simulink model "quad_6DOF_quaternion_ANSFT"  (R2023a)
settings: Solver=ode1  StartTime=0.0  StopTime=10  FixedStep=0.01  RelTol=1e-3
libraries: sharedtransform x5, simulink_extras x4, matrix_library x3, aerolibutil x3, simulink x3, sharedutil x2, robotcorelib x1, uavutilslib x1
settings Model: Creator=adan  LastModifiedBy=Adan Daniel

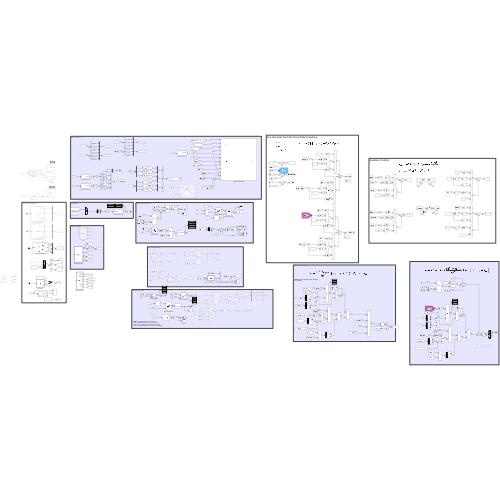
[thumbnail: Simulink's stored preview of the top-level diagram]
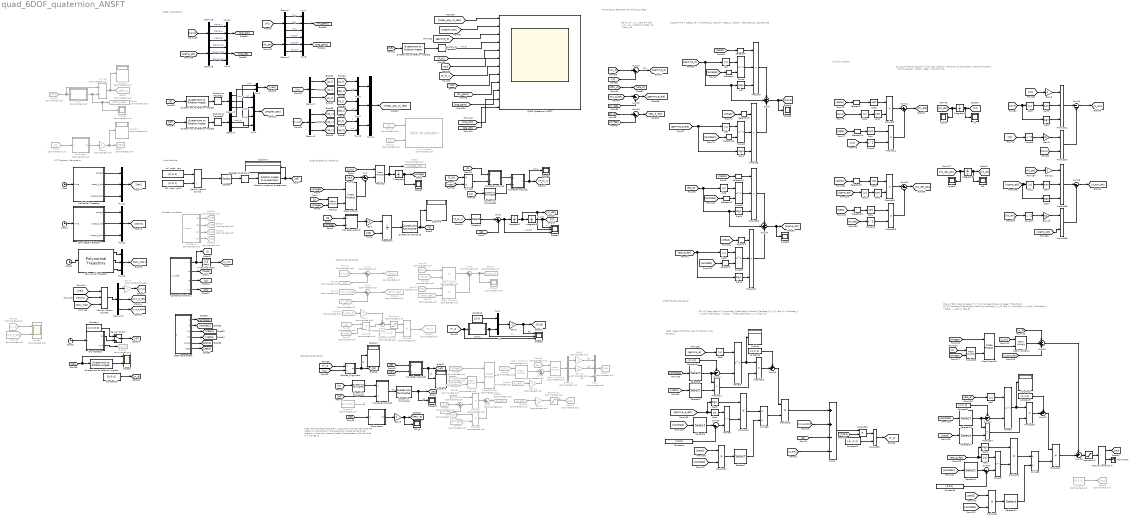
== system quad_6DOF_quaternion_ANSFT ==
  note: Note: It seems that the mass if missing in
      | the equation.
  note: ANSFT Position Controller
  note: $\tau = \Big [ \dot \omega_d + J^{-1} \omega \times J \omega + \frac{|\dot e|^{2-\lambda_2}\text{sign}(\dot e)}{\lambda_2 \xi_2} \Big (1 + \lambda_1 \xi_1|e|^{\lambda_1 - 1}\Big ) - u_{aux} \Big ]$
  note: $F_u = \frac{|\dot e|^{2-\lambda_2}\text{sign}(\dot e)}{\lambda_2 \xi_2} \Big (1 + \lambda_1 \xi_1|e|^{\lambda_1 - 1}\Big ) + \ddot \gamma_d - g - u_{aux}$
  note: Note : For the tilted Hexa-rotor I guess that I
      | have to calculate the vector nz, due to that in the
      | quad-rotor it used as the thrust direction in the body
      | frame of itself. Nonetheless in the FAH that will change ig
  note: Attitude PD Controller
  note: Initial attitude
  note: Constant variables
  note: Data Visualization
  note: Position PD Controller
  note: Quad Quaternion Modeling
  note: XYZ Trajectory Generation
  note: $e = x_d - x_1 \\ \dot e = \dot x_d - x_2 \\ \ddot e = \ddot x_d - \dot x_2$
  note: $\sigma = e + \zeta_1 |e| ^{\lambda_1} sign(e) + \zeta_2 | \dot e| ^{\lambda_2} sign(\dot e)$
  note: Non-Singular Fast Terminal Sliding Surface
  note: Auxiliary Control
  note: $u_{aux}=-2K(t) |\sigma|^{1/2} sign (\sigma) - \frac{K(t)^2}{2}\sigma \\ \dot K(t) = \alpha ^{1/2} |\sigma| ^{1/2} - \beta ^{1/2}K(t)^2$
  ANSFT parameters : MATLAB Function  TreatAsAtomicUnit=on
  Abs{,1..11} (12 alike) : Abs  SaturateOnIntegerOverflow=off
  Attitude_Alignment : Subsystem
  Clock{,1..3} (4 alike) : Clock
  Constant : Constant  Value=[1; 0; 0; 0]
  Constant1 : Constant  Value=[0; 0]
  Constant10 : Constant  Value=[0; 0; 0]
  Constant11 : Constant  Value=[-1; -1; 1]
  Constant2 : Constant  Commented=on  Value=[1; 0; 0; 0]
  Constant{3,5,7,9} (4 alike) : Constant  Value=[1; 1; 1]
  Constant4 : Constant  Value=[2;2;2]
  Constant6 : Constant  Commented=on  Value=[0; 0; 0]
  Constant8 : Constant  Value=[2;2;2]
  Constants Functions : MATLAB Function  TreatAsAtomicUnit=on
  Cross Product : matrix_library/Cross Product
  Cross Product1 : matrix_library/Cross Product
  Cross Product2 : matrix_library/Cross Product  Commented=on
  Degrees to Radians : simulink_extras/Transformations/Degrees to Radians
  Demux{1..4,6..9,11} (9 alike) : Demux  Outputs=3
  Demux5 : Demux  Commented=on  Outputs=3
  Display{,3..7} (6 alike) : Display
  Display1 : Display  Commented=on
  Display2 : Display  Commented=on
  Divide : Product  Commented=on  Inputs=*/
  Divide1 : Product  Inputs=*/
  Divide2 : Product  Inputs=*/
  Divide3 : Product  Inputs=*/
  Force adjustment : Constant  Commented=on  Value=[-1; -1; 1]
  From10 : From  Commented=on  GotoTag=PRP
  From12 : From  Commented=on  GotoTag=q
  From18 : From  Commented=on  GotoTag=xi
  From19 : From  Commented=on  GotoTag=kpt
  From20 : From  Commented=on  GotoTag=kdt
  From23 : From  Commented=on  GotoTag=xyz_d
  From24 : From  Commented=on  GotoTag=xyz_d_dot
  From26 : From  Commented=on  GotoTag=xi_dot
  From27 : From  Commented=on  GotoTag=xi
  From28 : From  Commented=on  GotoTag=error
  From29 : From  Commented=on  GotoTag=error_dot
  From30 : From  Commented=on  GotoTag=xyz_d
  From31 : From  Commented=on  GotoTag=g
  From44 : From  Commented=on  GotoTag=u_aux_z
  From46 : From  Commented=on  GotoTag=xyz_d_dot
  From47 : From  Commented=on  GotoTag=mass
  From56 : From  Commented=on  GotoTag=J_inv
  From57 : From  Commented=on  GotoTag=J
  From58 : From  Commented=on  GotoTag=omega
  From59 : From  Commented=on  GotoTag=omega
  From60 : From  Commented=on  GotoTag=PRV_e
  From61 : From  Commented=on  GotoTag=kdr
  From62 : From  Commented=on  GotoTag=omega
  From63 : From  Commented=on  GotoTag=kpr
  From64 : From  Commented=on  GotoTag=u_aux
  From65 : From  Commented=on  GotoTag=J
  From66 : From  Commented=on  GotoTag=u_aux
  From9 : From  Commented=on  GotoTag=q
  From90 : From  Commented=on  GotoTag=w_d
  Gain : Gain  Gain=0.5
  Gain1 : Gain  Commented=on  Gain=2
  Gain{4,7,9..11} (5 alike) : Gain  Commented=on  Gain=-1
  Gain12 : Gain  Gain=2
  Gain13 : Gain  Gain=0.5
  Gain2 : Gain  Gain=-1
  Gain3 : Gain  Gain=2
  Gain5 : Gain  Commented=through  Gain=0
  Gain6 : Gain  Gain=2
  Gain8 : Gain  Gain=0.5
  Goto13 : Goto  Commented=on  GotoTag=F_u
  Goto16 : Goto  Commented=on  GotoTag=kpt
  Goto17 : Goto  Commented=on  GotoTag=kdt
  Goto19 : Goto  Commented=on  GotoTag=kpr
  Goto20 : Goto  Commented=on  GotoTag=kdr
  Goto21 : Goto  Commented=on  GotoTag=error
  Goto22 : Goto  Commented=on  GotoTag=error_dot
  Goto29 : Goto  Commented=on  GotoTag=tau
  Goto3 : Goto  Commented=on  GotoTag=omega_dot
  Goto30 : Goto  Commented=on  GotoTag=u_aux
  Goto31 : Goto  Commented=on  GotoTag=u_aux_z
  Goto37 : Goto  Commented=on  GotoTag=tau
  Goto49 : Goto  Commented=on  GotoTag=w_d
  Goto59 : Goto  Commented=on  GotoTag=tau
  Goto6 : Goto  Commented=on  GotoTag=PRP
  Goto8 : Goto  Commented=on  GotoTag=PRP_u
  Goto9 : Goto  Commented=on  GotoTag=PRP_angle
  Helicoidal Trajectory : MATLAB Function  TreatAsAtomicUnit=on
  Integrator : Integrator  InitialCondition=[0; 0; 0]
  Integrator1 : Integrator  InitialConditionSource=external
  Integrator2 : Integrator  InitialCondition=[0; 0; 0]
  Integrator3 : Integrator  InitialCondition=[0; 0; 0]
  Integrator4 : Integrator  InitialCondition=[0;0;0]
  Integrator5 : Integrator  InitialCondition=[0;0;0]
  Invert 3x3 Matrix : aerolibutil/Invert  3x3 Matrix
  Kronecker product : Subsystem
  Kronecker product1 : Subsystem
  Kronecker product2 : Subsystem
  Kronecker product3 : Subsystem
  Kronecker product4 : Subsystem
  Kt : Scope
  Kt1 : Scope
  Kt_dot : Scope
  Kt_dot1 : Scope
  Lemniscate Trajectory : MATLAB Function  TreatAsAtomicUnit=on
  Manual Variant Sink : simulink/Signal Routing/Manual Variant Sink  NumChoices=2  LabelModeActiveChoice=V_1
  Manual Variant Source : simulink/Signal Routing/Manual Variant Source  NumChoices=2  LabelModeActiveChoice=V_1
  Manual Variant Source1 : simulink/Signal Routing/Manual Variant Source  NumChoices=3  LabelModeActiveChoice=V_3
  Manual Switch : ManualSwitch
  Matrix Multiply : Product  Commented=on
  Matrix Multiply1 : Product  Commented=on
  Matrix Multiply2 : Product  Multiplication=Matrix(*)
  Matrix Multiply3 : Product  Commented=on  Multiplication=Matrix(*)
  Matrix Multiply4 : Product  Commented=on  Multiplication=Matrix(*)
  Mux{1,3,8..10} (5 alike) : Mux  Inputs=2
  Mux{5..7,11..12,21..23} (8 alike) : Mux  Inputs=3
  Mux2 : Mux
  Mux4 : Mux  Commented=on  Inputs=3
  PD Gains : MATLAB Function  Commented=on  TreatAsAtomicUnit=on
  PRV_e : Scope
  Polynomial Trajectory : robotcorelib/Polynomial Trajectory  WaypointSource=Internal  Waypoints=[0, 0, 0, 0, 0, 0; 0, 0, 0, 0, 0, 0; 0, -2, -4, -4, -2, 0]*0  TimePoints=[ 0, 12, 24, 36, 48, 60]  TimeInterval=[ 1, 4 ]  Method=Cubic Polynomial  ParameterSource=Internal  VelocityBoundaryCondition=zeros( 3, 6)  AccelerationBoundaryCondition=zeros( 2, 5 )  SimulateUsing=Interpreted execution
  Power{,1,4..9} (8 alike) : Math  Operator=pow
  Power{2..3,10..11} (4 alike) : Math  Operator=square
  Product : Product  Multiplication=Matrix(*)
  Product1 : Product  Multiplication=Matrix(*)
  Product{9..11,13..18,20..25,28..29,31} (18 alike) : Product
  Product{4,8,12,26..27,30} (6 alike) : Product  Inputs=3
  Product19 : Product  Multiplication=Matrix(*)
  Product{2..3,6..7} (4 alike) : Product  Commented=on
  Product5 : Product  Commented=on  Multiplication=Matrix(*)
  QUAD Quaternion ANSFT : Scope  NumInputPorts=12
  Quaternion Conjugate : aerolibutil/Quaternion Conjugate
  Quaternion Conjugate2 : aerolibutil/Quaternion Conjugate
  Quaternion Normalize : sharedutil/Quaternion Normalize  aMode=aMode
  Quaternion Normalize1 : sharedutil/Quaternion Normalize  aMode=aMode
  Quaternions to Rotation Angles1 : sharedtransform/Quaternions to Rotation Angles  rotationOrder=ZYX  aMode=aMode
  Quaternions to Rotation Angles2 : sharedtransform/Quaternions to Rotation Angles  rotationOrder=XYZ  aMode=aMode
  Quaternions to Rotation Angles3 : sharedtransform/Quaternions to Rotation Angles  rotationOrder=ZYX  aMode=aMode
  Quaternions to Rotation Angles4 : sharedtransform/Quaternions to Rotation Angles  rotationOrder=ZYX  aMode=aMode
  Radians to Degrees1 : simulink_extras/Transformations/Radians to Degrees
  Radians to Degrees2 : simulink_extras/Transformations/Radians to Degrees
  Radians to Degrees3 : simulink_extras/Transformations/Radians to Degrees
  Rotation Angles to Quaternions : sharedtransform/Rotation Angles to Quaternions  rotationOrder=ZYX  aMode=aMode
  Saturation : Saturate  Commented=on  UpperLimit=[2; 2; 0]  LowerLimit=[-2; -2; -28]
  Saturation1 : Saturate  Commented=on
  Saturation2 : Saturate
  Scope : Scope  Commented=on
  Scope1 : Scope  NumInputPorts=2
  Scope{3,7..10} (5 alike) : Scope
  Scope2 : Scope  NumInputPorts=3
  Scope4 : Scope  NumInputPorts=3
  Scope5 : Scope  Commented=on
  Scope6 : Scope  Commented=on  NumInputPorts=2
  Selector : Selector  InputPortWidth=3  IndexOptions=Index vector (dialog)  Indices=[3 2 1]  OutputSizes=1
  Selector{1,3,10..14,18,20..21} (10 alike) : Selector  InputPortWidth=6  IndexOptions=Index vector (dialog)  Indices=[4:6]  OutputSizes=1
  Selector{4..9,15..17,19} (10 alike) : Selector  InputPortWidth=6  IndexOptions=Index vector (dialog)  Indices=[1:3]  OutputSizes=1
  Selector2 : Selector  InputPortWidth=4  IndexOptions=Index vector (dialog)  Indices=[2:4]  OutputSizes=1
  Sign{,1..7} (8 alike) : Signum
  Sqrt{,1..7} (8 alike) : Sqrt
  Subsystem : Subsystem  Commented=on
  Subsystem1 : Subsystem
  Sum{,11,14..16,25} (6 alike) : Sum  Inputs=|+-
  Sum1 : Sum  Inputs=|++
  Sum10 : Sum  Inputs=|-+
  Sum12 : Sum  Inputs=|--
  Sum13 : Sum  Commented=on  Inputs=|+-
  Sum17 : Sum  Inputs=-+|
  Sum18 : Sum  Inputs=++|
  Sum19 : Sum  Inputs=++-
  Sum2 : Sum  Commented=on  Inputs=|+-
  Sum20 : Sum  Inputs=|-+
  Sum21 : Sum  Inputs=-+|
  Sum22 : Sum  Inputs=++|
  Sum23 : Sum  Inputs=++|
  Sum24 : Sum  Inputs=+++
  Sum26 : Sum  Inputs=|--
  Sum3 : Sum  Commented=on  Inputs=|+-
  Sum4 : Sum  Commented=on  Inputs=|++
  Sum5 : Sum  Commented=on  Inputs=+-|
  Sum6 : Sum  Inputs=++--
  Sum7 : Sum  Commented=on  Inputs=|++
  Sum8 : Sum  Commented=on  Inputs=|++
  Sum9 : Sum  Inputs=+++
  Terminator : Terminator
  UAV Animation : uavutilslib/UAV Animation  Commented=on  UAVType=Multirotor  UAVSize=1  InertialZDirection=Down  SampleTime=-1
  Yaw trajectory : MATLAB Function  TreatAsAtomicUnit=on
  norm : MATLAB Function  Commented=on  TreatAsAtomicUnit=on
  norm1 : MATLAB Function  TreatAsAtomicUnit=on
  "roll, pitch, yaw" : Constant  Value=[5; 0; 0]
  "roll, pitch, yaw1" : Constant  Value=[0; 0; 1]
  wires:
  Constants Functions/1(J) -> [J], Invert 3x3 Matrix/1
  Invert 3x3 Matrix/1 -> [J_inv]
  [tau] -> Sum/1
  [J] -> Product/1
  [omega] -> Product/2
  [omega] -> Cross Product/1
  Product/1 -> Cross Product/2
  Cross Product/1 -> Sum/2
  Sum/1 -> Product1/2
  [J_inv] -> Product1/1
  Product1/1 -> Goto3/1, Integrator/1
  Integrator/1 -> Scope7/1, [omega]
  [omega] -> Kronecker product/2(p)
  Kronecker product/1(r) -> Gain/1
  Gain/1 -> Integrator1/1
  Degrees to Radians/1 -> Rotation Angles to Quaternions/1
  Selector/1 -> Degrees to Radians/1
  Rotation Angles to Quaternions/1 -> Display4/1, [q0]
  [q0] -> Integrator1/2
  Integrator1/1 -> Quaternion Normalize/1
  [q] -> Kronecker product/1(q)
  Quaternion Normalize/1 -> Display5/1, [q]
  From12/1 -> UAV Animation/2
  From18/1 -> UAV Animation/1
  Constants Functions/2(m) -> [mass]
  From9/1 -> Subsystem/1(q)
  Subsystem/1(lnq) -> Gain1/1
  Gain1/1 -> Display1/1, Goto6/1
  From10/1 -> norm/1(u), Divide/1
  norm/1(y) -> Scope/1, Goto9/1, Divide/2
  Divide/1 -> Goto8/1, Display2/1
  Constants Functions/3(g) -> [g]
  Kronecker product1/1(r) -> Kronecker product2/1(q)
  Kronecker product2/1(r) -> Scope3/1, [F_th_I]  "f_th_I"
  [F_th_I] -> Selector2/1
  [mass] -> Divide1/2
  Selector2/1 -> Sum1/1
  [g] -> Sum1/2
  Sum1/1 -> Scope4/3, Integrator2/1  "x_ddot"
  Integrator2/1 -> Scope4/2, [xi_dot], Integrator3/1  "x_dot"
  Integrator3/1 -> Scope4/1, [xi]  "x"
  PD Gains/1(kpt) -> Goto16/1
  PD Gains/2(kdt) -> Goto17/1
  PD Gains/4(kdr) -> Goto20/1
  PD Gains/3(kpr) -> Goto19/1
  Polynomial Trajectory/3 -> Mux23/3
  Mux22/1 -> [lemni]
  Clock1/1 -> Polynomial Trajectory/1
  Manual Variant Source1/1 -> Demux11/1
  Demux11/2 -> [xyz_d_dot]
  Mux21/1 -> [heli]
  Helicoidal Trajectory/1(pose_d) -> Mux21/1
  Lemniscate Trajectory/2(pose_d_dot) -> Mux22/2
  [lemni] -> Manual Variant Source1/2
  Clock2/1 -> Lemniscate Trajectory/1(time)
  [poly_tray] -> Manual Variant Source1/3
  Helicoidal Trajectory/3(pose_d_ddot) -> Mux21/3
  [heli] -> Manual Variant Source1/1
  Lemniscate Trajectory/3(pose_d_ddot) -> Mux22/3
  Mux23/1 -> [poly_tray]
  Clock/1 -> Helicoidal Trajectory/1(time)
  Polynomial Trajectory/2 -> Mux23/2
  Polynomial Trajectory/1 -> Mux23/1
  Helicoidal Trajectory/2(pose_d_dot) -> Mux21/2
  Demux11/3 -> [xyz_d_ddot]
  Demux11/1 -> Gain5/1
  Lemniscate Trajectory/1(pose_d) -> Mux22/1
  From23/1 -> Sum2/1
  From27/1 -> Sum2/2
  From24/1 -> Sum3/1
  From26/1 -> Sum3/2
  Sum2/1 -> Goto21/1
  Sum3/1 -> Goto22/1
  From19/1 -> Matrix Multiply/1
  From28/1 -> Matrix Multiply/2
  From20/1 -> Matrix Multiply1/1
  From29/1 -> Matrix Multiply1/2
  Matrix Multiply/1 -> Sum4/1
  Matrix Multiply1/1 -> Sum4/2
  Sum5/1 -> Saturation/1
  [F_u] -> norm1/1(u), Scope2/3  "fu"
  norm1/1(y) -> Mux1/2, Scope2/2  "nu"
  Constant1/1 -> Mux1/1
  Mux1/1 -> Gain2/1
  Gain2/1 -> [F_th], Scope2/1  "fth"
  [angular_pos] -> QUAD Quaternion ANSFT/2
  [gamma_e] -> QUAD Quaternion ANSFT/3
  Quaternions to Rotation Angles2/1 -> Radians to Degrees2/1
  [F_th_I] -> QUAD Quaternion ANSFT/7
  [yaw] -> QUAD Quaternion ANSFT/8
  [tau] -> QUAD Quaternion ANSFT/6
  [F_th] -> QUAD Quaternion ANSFT/5
  [linear_pos_vs_des] -> QUAD Quaternion ANSFT/1
  [q_x] -> Mux8/1  "x"
  [qd_y] -> Mux9/2  "y_d"
  Mux8/1 -> Mux11/1
  Mux9/1 -> Mux11/2
  [qd_x] -> Mux8/2  "x_d"
  Mux11/1 -> [linear_pos_vs_des]
  [q_y] -> Mux9/1  "y"
  Mux10/1 -> Mux11/3
  [qd_z] -> Mux10/2  "z_d"
  [q_z] -> Mux10/1  "z"
  Demux6/3 -> [qd_z]
  [xyz_d] -> Demux6/1
  Demux6/2 -> [qd_y]
  Demux6/1 -> [qd_x]
  Demux2/1 -> [q_x]
  Demux2/2 -> [q_y]
  Demux2/3 -> [q_z]
  [xi] -> Demux2/1
  [q] -> Quaternions to Rotation Angles1/1
  Subsystem1/1(lnq) -> Gain3/1
  Clock3/1 -> Yaw trajectory/1(t)
  [qz] -> Kronecker product3/2(p)
  Kronecker product3/1(r) -> Display6/1, [qd]  "qd"
  [q] -> Quaternion Conjugate/1
  Quaternion Conjugate/1 -> Kronecker product4/1(q)
  Kronecker product4/1(r) -> Quaternion Normalize1/1  "qe"
  Gain3/1 -> PRV_e/1, [PRV_e]
  Constants Functions/4(nz) -> [nz]
  [F_u] -> Attitude_Alignment/1(nu)
  [nz] -> Attitude_Alignment/2(nz)
  Attitude_Alignment/1(qt) -> Display7/1, [qt]  "qt"
  [qe] -> Quaternions to Rotation Angles2/1
  [qd] -> Quaternions to Rotation Angles3/1
  Quaternions to Rotation Angles1/1 -> Radians to Degrees1/1
  Demux3/1 -> Mux3/1  "yaw"
  Demux3/2 -> Mux2/3  "pitch"
  Demux3/3 -> Mux2/1  "roll"
  Demux4/1 -> Mux3/2  "yaw_d"
  Demux4/3 -> Mux2/2  "roll_d"
  Demux4/2 -> Mux2/4  "pitch_d"
  Quaternions to Rotation Angles3/1 -> Radians to Degrees3/1
  [qz] -> Scope1/1, Quaternions to Rotation Angles4/1
  Quaternions to Rotation Angles4/1 -> Scope1/2
  Yaw trajectory/1(qz) -> Manual Switch/2
  Constant/1 -> Manual Switch/1
  Manual Switch/1 -> [qz]
  From58/1 -> Product5/2
  Product5/1 -> Cross Product2/2
  From57/1 -> Product5/1
  From59/1 -> Cross Product2/1
  Cross Product2/1 -> Matrix Multiply3/2
  From56/1 -> Matrix Multiply3/1
  From62/1 -> Sum13/2
  From61/1 -> Product7/1
  Product7/1 -> Sum7/1
  From63/1 -> Product6/1
  From60/1 -> Product6/2
  Product6/1 -> Sum7/2
  Sum7/1 -> Goto30/1
  Matrix Multiply3/1 -> Sum8/1
  From64/1 -> Gain11/1
  Sum8/1 -> Matrix Multiply4/2
  From65/1 -> Matrix Multiply4/1
  Matrix Multiply4/1 -> Demux5/1
  Mux2/1 -> [angular_pos]
  Radians to Degrees2/1 -> QUAD Quaternion ANSFT/4  "rpy_e"
  Sum4/1 -> Scope5/1, Goto31/1
  From44/1 -> Gain4/1
  Radians to Degrees1/1 -> Demux3/1
  Radians to Degrees3/1 -> Demux4/1
  [qe] -> Subsystem1/1(q)
  Saturation/1 -> Product3/1
  Gain4/1 -> Sum5/1
  [q] -> Quaternion Conjugate2/1
  [q] -> Kronecker product1/1(q)
  From30/1 -> Scope6/1
  From46/1 -> Scope6/2
  Product2/1 -> Sum5/2
  From31/1 -> Product2/1
  From47/1 -> Product2/2
  Gain5/1 -> [xyz_d]
  [F_th] -> Divide1/1
  [qd] -> Kronecker product4/2(p)
  From66/1 -> Gain7/1
  Quaternion Conjugate2/1 -> Kronecker product2/2(p)
  Manual Variant Source/1 -> Selector/1
  "roll, pitch, yaw"/1 -> Manual Variant Source/1
  "roll, pitch, yaw1"/1 -> Manual Variant Source/2
  Saturation1/1 -> Goto37/1  "tau"
  Force adjustment/1 -> Product3/2
  Product3/1 -> Goto13/1
  Gain7/1 -> Saturation1/1
  Quaternion Normalize1/1 -> Scope10/1, [qe]  "qe"
  Mux3/1 -> [yaw]
  [zeta1] -> Selector4/1
  Sign/1 -> Product4/3
  Power1/1 -> Product8/2
  [gamma_e] -> Sum9/2, Sign/1, Abs/1
  Product8/1 -> Sum9/3
  Abs1/1 -> Power1/1
  [zeta2] -> Selector15/1
  Sign1/1 -> Product8/3
  [lambda1] -> Selector5/1
  [lambda2] -> Selector16/1
  Power/1 -> Product4/2
  Sum9/1 -> Scope9/1, [sigma]
  Product4/1 -> Sum9/1
  [gamma_e_dot] -> Sign1/1, Abs1/1
  Abs/1 -> Power/1
  Power2/1 -> Product11/2
  Product10/1 -> Sum12/2
  [Kt] -> Gain6/1
  Power3/1 -> Gain8/1
  Sum11/1 -> [Kt_dot]
  Product9/1 -> Sum11/1
  [Kt_dot] -> Kt_dot/1, Integrator4/1
  [sigma] -> Sign2/1, Abs3/1
  [alpha] -> Selector17/1
  Sqrt/1 -> Product11/1
  Sqrt1/1 -> Product9/1
  [Kt] -> Power2/1
  [beta] -> Selector19/1
  Product11/1 -> Sum11/2
  Gain6/1 -> Product12/1
  Abs3/1 -> Sqrt3/1
  Abs2/1 -> Sqrt2/1
  [Kt] -> Power3/1
  Gain8/1 -> Product10/1
  Sign2/1 -> Product12/3
  Sqrt2/1 -> Product9/2
  Sqrt3/1 -> Product12/2
  Sum12/1 -> [u_aux]
  Product12/1 -> Sum12/1
  [sigma] -> Product10/2
  Integrator4/1 -> Kt/1, [Kt]
  Divide1/1 -> Kronecker product1/2(p)
  [qt] -> Kronecker product3/1(q)
  Demux5/1 -> Gain9/1
  Gain9/1 -> Mux4/1  "t_x"
  Demux5/2 -> Gain10/1
  Demux5/3 -> Mux4/3  "t_z"
  Mux4/1 -> Goto29/1
  Gain10/1 -> Mux4/2  "t_y"
  Gain11/1 -> Sum8/2
  Yaw trajectory/2(w_d) -> Goto49/1
  From90/1 -> Sum13/1
  Sum13/1 -> Product7/2
  [xi] -> Sum14/2
  [w_d] -> Sum16/1
  [xi_dot] -> Sum15/2
  [omega] -> Sum16/2
  [xyz_d] -> Sum14/1
  [xyz_d_dot] -> Sum15/1
  ANSFT parameters/1(lambda1) -> [lambda1]
  ANSFT parameters/4(xi2) -> [zeta2]
  ANSFT parameters/2(lambda2) -> [lambda2]
  ANSFT parameters/3(xi1) -> [zeta1]
  ANSFT parameters/6(beta) -> [beta]
  ANSFT parameters/5(alpha) -> [alpha]
  [xyz_d_ddot] -> Sum6/2
  [g] -> Sum6/3
  [u_aux] -> Sum6/4
  [gamma_e_dot] -> Sign3/1, Abs4/1
  [lambda2] -> Selector6/1
  Constant4/1 -> Sum10/2
  Sum10/1 -> Power4/2
  Abs4/1 -> Power4/1
  Selector6/1 -> Sum10/1
  Sign3/1 -> Product13/1
  Power4/1 -> Product13/2
  Product13/1 -> Divide2/1
  [lambda2] -> Product14/2
  [zeta2] -> Product14/1
  Product14/1 -> Selector7/1
  Selector7/1 -> Divide2/2
  Divide2/1 -> Product15/2
  [gamma_e] -> Abs5/1
  Abs5/1 -> Power5/1
  Sum17/1 -> Power5/2
  [lambda1] -> Selector8/1
  Selector8/1 -> Product17/1, Sum17/2
  Constant3/1 -> Sum17/1
  Power5/1 -> Display/1, Product16/1
  Selector9/1 -> Product17/2
  [zeta1] -> Selector9/1
  Product17/1 -> Product16/2
  Sum18/1 -> Product15/1
  Product16/1 -> Sum18/2
  Constant5/1 -> Sum18/1
  Product15/1 -> Sum6/1
  Constant6/1 -> Goto59/1
  Constant2/1 -> ?
  Sum6/1 -> Product18/1
  [Kt] -> Demux7/1
  Mux7/1 -> [lin_gains]
  Demux7/3 -> Mux7/3  "Kt_z"
  Demux7/2 -> Mux7/2  "Kt_y"
  Demux7/1 -> Mux7/1  "Kt_x"
  [lin_gains] -> QUAD Quaternion ANSFT/9
  [ang_gains] -> QUAD Quaternion ANSFT/10
  [mass] -> Product18/2
  [J] -> Product19/1
  Cross Product1/1 -> Matrix Multiply2/2
  [omega] -> Cross Product1/1
  [J_inv] -> Matrix Multiply2/1
  [omega] -> Product19/2
  Product19/1 -> Cross Product1/2
  Matrix Multiply2/1 -> Sum19/2
  [u_aux_att] -> Sum19/3
  [w_d] -> Sum19/1
  Selector14/1 -> Product24/2
  Power6/1 -> Product20/2
  Constant7/1 -> Sum21/1
  Product21/1 -> Selector12/1
  [lambda2] -> Product21/2
  Product23/1 -> Sum22/2
  Selector12/1 -> Divide3/2
  [zeta1] -> Selector14/1
  Product20/1 -> Divide3/1
  Constant9/1 -> Sum22/1
  Sum21/1 -> Power7/2
  Sum22/1 -> Product22/1
  [lambda2] -> Selector11/1
  Sign4/1 -> Product20/1
  Sum20/1 -> Power6/2
  Selector11/1 -> Sum20/1
  Constant8/1 -> Sum20/2
  [zeta2] -> Product21/1
  Power7/1 -> Display3/1, Product23/1
  Abs7/1 -> Power7/1
  Selector13/1 -> Product24/1, Sum21/2
  [lambda1] -> Selector13/1
  Abs6/1 -> Power6/1
  [eta_e] -> Abs7/1
  Product24/1 -> Product23/2
  [eta_e_dot] -> Sign4/1, Abs6/1
  Divide3/1 -> Product22/2
  Product22/1 -> Sum23/2
  Sum23/1 -> Saturation2/1
  Sum19/1 -> Sum23/1
  Constant10/1 -> [w_d]
  Product18/1 -> Product25/1
  Constant11/1 -> Product25/2
  Product25/1 -> [F_u]
  Saturation2/1 -> Manual Variant Sink/1
  Manual Variant Sink/1 -> [tau]
  Manual Variant Sink/2 -> Terminator/1
  Sum15/1 -> [gamma_e_dot]
  Sum14/1 -> [gamma_e]  "des"
  Sum16/1 -> [eta_e_dot]
  [PRV_e] -> [eta_e]
  Selector4/1 -> Product4/1
  Selector5/1 -> Power/2
  Selector15/1 -> Product8/1
  Selector16/1 -> Power1/2
  Selector17/1 -> Sqrt1/1
  [sigma] -> Abs2/1
  Selector19/1 -> Sqrt/1
  Selector18/1 -> Power8/2
  Selector10/1 -> Product26/1
  Selector3/1 -> Power9/2
  Product26/1 -> Sum24/1
  Abs8/1 -> Power8/1
  Power9/1 -> Product27/2
  Power8/1 -> Product26/2
  [eta_e_dot] -> Abs9/1, Sign6/1
  [eta_e] -> Sum24/2, Sign5/1, Abs8/1
  Selector1/1 -> Product27/1
  [lambda1] -> Selector18/1
  Sign6/1 -> Product27/3
  Abs9/1 -> Power9/1
  Product27/1 -> Sum24/3
  Sign5/1 -> Product26/3
  Sum24/1 -> Scope8/1, [sigma_att]
  [lambda2] -> Selector3/1
  [zeta2] -> Selector1/1
  [zeta1] -> Selector10/1
  Selector21/1 -> Sqrt4/1
  Product30/1 -> Sum26/1
  Sqrt7/1 -> Product30/2
  Sqrt4/1 -> Product29/1
  Selector20/1 -> Sqrt5/1
  [sigma_att] -> Sign7/1, Abs11/1
  [beta] -> Selector21/1
  [Kt_att] -> Power10/1
  Sign7/1 -> Product30/3
  [sigma_att] -> Abs10/1
  Gain13/1 -> Product28/1
  Integrator5/1 -> Kt1/1, [Kt_att]
  Abs10/1 -> Sqrt6/1
  Power11/1 -> Gain13/1
  Product28/1 -> Sum26/2
  Power10/1 -> Product29/2
  [alpha] -> Selector20/1
  Product31/1 -> Sum25/1
  Sqrt5/1 -> Product31/1
  [Kt_att] -> Power11/1
  [sigma_att] -> Product28/2
  Sqrt6/1 -> Product31/2
  Product29/1 -> Sum25/2
  [Kt_dot_att] -> Kt_dot1/1, Integrator5/1
  Abs11/1 -> Sqrt7/1
  Sum26/1 -> [u_aux_att]
  Sum25/1 -> [Kt_dot_att]
  [Kt_att] -> Gain12/1
  Gain12/1 -> Product30/1
  Demux1/2 -> Mux5/2  "Kt_pitch"
  Demux1/3 -> Mux5/3  "Kt_yaw"
  Mux5/1 -> [ang_gains]
  Demux1/1 -> Mux5/1  "Kt_roll"
  [Kt_att] -> Demux1/1
  Demux8/2 -> Mux6/2  "sigma_pitch"
  Demux8/3 -> Mux6/3  "sigma_yaw"
  [sigma_att] -> Demux8/1
  Demux9/2 -> Mux12/2  "sigma_y"
  Demux9/3 -> Mux12/3  "sigma_z"
  Demux9/1 -> Mux12/1  "sigma_x"
  Demux8/1 -> Mux6/1  "sigma_roll"
  [sigma] -> Demux9/1
  Mux12/1 -> [sig_pos]
  Mux6/1 -> [sig_att]
  [sig_pos] -> QUAD Quaternion ANSFT/11
  [sig_att] -> QUAD Quaternion ANSFT/12

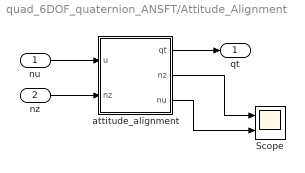
== system quad_6DOF_quaternion_ANSFT/Attitude_Alignment ==
  nu : Inport
  nz : Inport  Port=2
  Scope : Scope  NumInputPorts=2
  attitude_alignment : MATLAB Function  TreatAsAtomicUnit=on
  qt : Outport
  wires:
  attitude_alignment/1(qt) -> qt/1
  nz/1 -> attitude_alignment/2("nz ")
  nu/1 -> attitude_alignment/1(u)
  attitude_alignment/2(nz) -> Scope/1
  attitude_alignment/3(nu) -> Scope/2

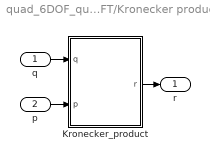
== system quad_6DOF_quaternion_ANSFT/Kronecker product ==
  q : Inport
  p : Inport  Port=2
  Kronecker_product : MATLAB Function  TreatAsAtomicUnit=on
  r : Outport
  wires:
  q/1 -> Kronecker_product/1(q)
  p/1 -> Kronecker_product/2(p)
  Kronecker_product/1(r) -> r/1

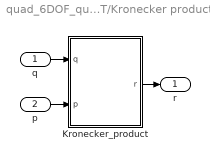
== system quad_6DOF_quaternion_ANSFT/Kronecker product1 ==
  q : Inport
  p : Inport  Port=2
  Kronecker_product : MATLAB Function  TreatAsAtomicUnit=on
  r : Outport
  wires:
  q/1 -> Kronecker_product/1(q)
  p/1 -> Kronecker_product/2(p)
  Kronecker_product/1(r) -> r/1

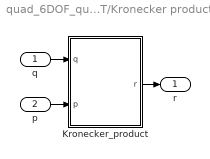
== system quad_6DOF_quaternion_ANSFT/Kronecker product2 ==
  q : Inport
  p : Inport  Port=2
  Kronecker_product : MATLAB Function  TreatAsAtomicUnit=on
  r : Outport
  wires:
  q/1 -> Kronecker_product/1(q)
  p/1 -> Kronecker_product/2(p)
  Kronecker_product/1(r) -> r/1

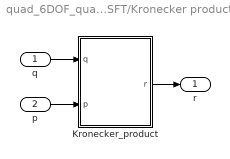
== system quad_6DOF_quaternion_ANSFT/Kronecker product3 ==
  q : Inport
  p : Inport  Port=2
  Kronecker_product : MATLAB Function  TreatAsAtomicUnit=on
  r : Outport
  wires:
  q/1 -> Kronecker_product/1(q)
  p/1 -> Kronecker_product/2(p)
  Kronecker_product/1(r) -> r/1

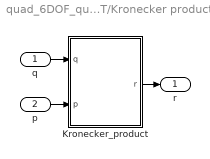
== system quad_6DOF_quaternion_ANSFT/Kronecker product4 ==
  q : Inport
  p : Inport  Port=2
  Kronecker_product : MATLAB Function  TreatAsAtomicUnit=on
  r : Outport
  wires:
  q/1 -> Kronecker_product/1(q)
  p/1 -> Kronecker_product/2(p)
  Kronecker_product/1(r) -> r/1

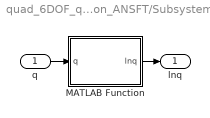
== system quad_6DOF_quaternion_ANSFT/Subsystem ==
  q : Inport
  MATLAB Function : MATLAB Function  TreatAsAtomicUnit=on
  lnq : Outport
  wires:
  MATLAB Function/1(lnq) -> lnq/1
  q/1 -> MATLAB Function/1(q)

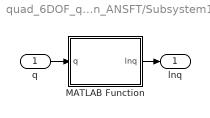
== system quad_6DOF_quaternion_ANSFT/Subsystem1 ==
  q : Inport
  MATLAB Function : MATLAB Function  TreatAsAtomicUnit=on
  lnq : Outport
  wires:
  MATLAB Function/1(lnq) -> lnq/1
  q/1 -> MATLAB Function/1(q)

== matlab function quad_6DOF_quaternion_ANSFT/norm1 ==
  data: u input; y output
function y = fcn(u)

y = norm(u);

== matlab function quad_6DOF_quaternion_ANSFT/Attitude_Alignment/attitude_alignment ==
  data: u input; qt output size=[4 1]; nz input; nz output; nu output
function [qt, nz, nu] = fcn(u, nz)

% qt = zeros(4, 1);
% normalize vector
nu = - u / norm(u);
nz = nz / norm(nz);

% vector properties

% attitude alignment
% if thrust is aligned with body frame z-axis, return a 0 quaternion
if cross(nu, nz) == zeros(3, 1)
    qt = [1; 0; 0; 0];
else
    qt = [sqrt((1 + dot(nu, nz))/(2));
          ((cross(nu, nz))/(norm(cross(nu, nz)))) * sqrt((1 - dot(nu, nz))/(2))];
    % for j = 1:1:length(qt)
    %     if qt(j) < 0
    %         qt = dot(qt, [-1; 1; 1; 1]);
    %     end
    % end
end

== matlab function quad_6DOF_quaternion_ANSFT/Kronecker product3/Kronecker_product ==
  data: q input; r output size=[4 1]; p input
function r = fcn(q, p)

%{
    Function to describe in matrix math the Kronecker product between
    two quaternions
    
    r = p kronecker q
    %}

    len = length(p);

    % if 

    if len == 3 && length(q) == 4
        p1 = [0; p];
        q0 = q(1);
        q1 = q(2);
        q2 = q(3);
        q3 = q(4);
        
        % skew symmetric matrix
        q_matrix = [q0, -q1, -q2, -q3;
                  q1, q0, -q3, q2;
                  q2, q3, q0, -q1;
                  q3, -q2, q1, q0];
        
        r = q_matrix * p1;

    elseif len == 4
        q0 = q(1);
        q1 = q(2);
        q2 = q(3);
        q3 = q(4);
        
        % skew symmetric matrix
        q_matrix = [q0, -q1, -q2, -q3;
                  q1, q0, -q3, q2;
                  q2, q3, q0, -q1;
                  q3, -q2, q1, q0];
        
        r = q_matrix * p;

    else
        error('Quaternions dimensions do not match')
    end

== matlab function quad_6DOF_quaternion_ANSFT/Subsystem1/MATLAB Function ==
  data: q input; lnq output size=[3 1]
function lnq = fcn(q)

if length(q) == 4
    q0 = q(1);
    q_vec = [q(2); q(3); q(4)];

    if norm(q_vec) == 0
        lnq = [0; 0; 0];
    else
        % q0 = real(q0);
        lnq = (q_vec / (norm(q_vec)) ) * acos(q0);
    end
else
    error('Input must be a vector 4 by 1 (Quaternion)')
end

== matlab function quad_6DOF_quaternion_ANSFT/Yaw trajectory ==
  data: t input; qz output; w_d output
function [qz, w_d] = fcn(t)

if t < 5
    yaw = 0;
    w_d = [0; 0; 0];
else
    yaw = 0.2*(t - 5);
    w_d = [0; 0; 0.2];
end
qz = [cos(yaw/2);
      0;
      0;
      sin(yaw/2)];

== matlab function quad_6DOF_quaternion_ANSFT/Kronecker product4/Kronecker_product ==
  data: q input; r output size=[4 1]; p input
function r = fcn(q, p)

%{
    Function to describe in matrix math the Kronecker product between
    two quaternions
    
    r = p kronecker q
    %}

    len = length(p);

    if len == 3 && length(q) == 4
        p1 = [0; p];
        q0 = q(1);
        q1 = q(2);
        q2 = q(3);
        q3 = q(4);
        
        % skew symmetric matrix
        q_matrix = [q0, -q1, -q2, -q3;
                  q1, q0, -q3, q2;
                  q2, q3, q0, -q1;
                  q3, -q2, q1, q0];
        
        r = q_matrix * p1;

    elseif len == 4
        q0 = q(1);
        q1 = q(2);
        q2 = q(3);
        q3 = q(4);
        
        % skew symmetric matrix
        q_matrix = [q0, -q1, -q2, -q3;
                  q1, q0, -q3, q2;
                  q2, q3, q0, -q1;
                  q3, -q2, q1, q0];
        
        r = q_matrix * p;

    else
        error('Quaternions dimensions do not match')
    end

== matlab function quad_6DOF_quaternion_ANSFT/ANSFT parameters ==
  data: lambda1 output; unused input; lambda2 output; xi1 output; xi2 output; alpha output; beta output
function [lambda1, lambda2, xi1, xi2, alpha, beta]= fcn(~)

xi1 = [1.5; 0.25; 0.01; 7.5; 8; 2.5];

xi2 = [13; 5; 5; 3.75; 05; 10];

lambda1 = [2; 2; 2; 3; 2.5; 5];

lambda2 = [1.3; 1.35; 1.3; 1.5; 1.3; 1.5];

alpha = [0.05; 0.075; 0.05; 1.25; 10; 0.05];

beta = [15; 5; 5; 1; 0.05; 0.01];

== matlab function quad_6DOF_quaternion_ANSFT/Subsystem/MATLAB Function ==
  data: q input; lnq output size=[3 1]
function lnq = fcn(q)

if length(q) == 4
    q0 = q(1);
    
    q_vec = [q(2); q(3); q(4)];

    if norm(q_vec) == 0
        lnq = [0; 0; 0];
    else
        lnq = (q_vec / (norm(q_vec)) ) * acos(q0);
    end
else
    error('Input must be a vector 4 by 1 (Quaternion)')
end

== matlab function quad_6DOF_quaternion_ANSFT/Kronecker product/Kronecker_product ==
  data: q input; r output size=[4 1]; p input
function r = fcn(q, p)

%{
    Function to describe in matrix math the Kronecker product between
    two quaternions
    
    r = p kronecker q
    %}

    len = length(p);

    if len == 3 && length(q) == 4
        p1 = [0; p];
        q0 = q(1);
        q1 = q(2);
        q2 = q(3);
        q3 = q(4);
        
        % skew symmetric matrix
        q_matrix = [q0, -q1, -q2, -q3;
                  q1, q0, -q3, q2;
                  q2, q3, q0, -q1;
                  q3, -q2, q1, q0];
        
        r = q_matrix * p1;

    elseif len == 4
        q0 = q(1);
        q1 = q(2);
        q2 = q(3);
        q3 = q(4);
        
        % skew symmetric matrix
        q_matrix = [q0, -q1, -q2, -q3;
                  q1, q0, -q3, q2;
                  q2, q3, q0, -q1;
                  q3, -q2, q1, q0];
        
        r = q_matrix * p;

    else
        error('Quaternions dimensions do not match')
    end

== matlab function quad_6DOF_quaternion_ANSFT/Constants Functions ==
  data: unused input; J output; m output; g output; nz output
function [J, m, g, nz] = fcn(~)

m = 2.0; % kg

Jxx =  0.0411; % kg m²
Jyy = 0.0478; % kg m²
Jzz = 0.0599; % kg m²

J = [Jxx, 0, 0;
     0, Jyy, 0;
     0, 0, Jzz];

g = [0; 0; 9.81];

nz = [0; 0; 1];

== matlab function quad_6DOF_quaternion_ANSFT/norm ==
  data: u input; y output
function y = fcn(u)

y = norm(u);

== matlab function quad_6DOF_quaternion_ANSFT/Kronecker product1/Kronecker_product ==
  data: q input; r output; p input
function r = fcn(q, p)

%{
    Function to describe in matrix math the Kronecker product between
    two quaternions
    
    r = p kronecker q
    %}

    len = length(p);

    if len == 3
        p1 = [0; p];
        q0 = q(1);
        q1 = q(2);
        q2 = q(3);
        q3 = q(4);
        
        % skew symmetric matrix
        q_matrix = [q0, -q1, -q2, -q3;
                  q1, q0, -q3, q2;
                  q2, q3, q0, -q1;
                  q3, -q2, q1, q0];
        
        r = q_matrix * p1;

    elseif len == 4
        q0 = q(1);
        q1 = q(2);
        q2 = q(3);
        q3 = q(4);
        
        % skew symmetric matrix
        q_matrix = [q0, -q1, -q2, -q3;
                  q1, q0, -q3, q2;
                  q2, q3, q0, -q1;
                  q3, -q2, q1, q0];
        
        r = q_matrix * p;

    else
        error('Quaternions dimensions do not match')
    end

== matlab function quad_6DOF_quaternion_ANSFT/Kronecker product2/Kronecker_product ==
  data: q input; r output; p input
function r = fcn(q, p)

%{
    Function to describe in matrix math the Kronecker product between
    two quaternions
    
    r = p kronecker q
    %}

    len = length(p);

    if len == 3
        p1 = [0; p];
        q0 = q(1);
        q1 = q(2);
        q2 = q(3);
        q3 = q(4);
        
        % skew symmetric matrix
        q_matrix = [q0, -q1, -q2, -q3;
                  q1, q0, -q3, q2;
                  q2, q3, q0, -q1;
                  q3, -q2, q1, q0];
        
        r = q_matrix * p1;

    elseif len == 4
        q0 = q(1);
        q1 = q(2);
        q2 = q(3);
        q3 = q(4);
        
        % skew symmetric matrix
        q_matrix = [q0, -q1, -q2, -q3;
                  q1, q0, -q3, q2;
                  q2, q3, q0, -q1;
                  q3, -q2, q1, q0];
        
        r = q_matrix * p;

    else
        error('Quaternions dimensions do not match')
    end

== matlab function quad_6DOF_quaternion_ANSFT/PD Gains ==
  data: unused input; kpt output; kdt output; kpr output; kdr output
function [kpt, kdt, kpr, kdr] = fcn(~)

kpt = [1.5; 1.5; 8];
kdt = [2.75; 2.75; 4];
kpr = [15; 15; 10];
kdr = [5; 5; 5];

== matlab function quad_6DOF_quaternion_ANSFT/Helicoidal Trajectory ==
  data: time input; pose_d output; pose_d_dot output; pose_d_ddot output
function [pose_d, pose_d_dot, pose_d_ddot]= fcn(time)

pos_z = time / 12;
f = 0.15;
arg = f * (time - 5);
r = 2;

% hover for 5 s | include inclination in roll
% 5 metros al menos

if (time < 5)
    pos_x = 0;
    pos_y = 0;
    % roll = 0;
else
    pos_x = -2 + r * cos (arg);
    pos_y = r * sin (arg);
    % roll = 0.15;
end

% roll = 0;
% yaw = time * 0;

pose_d = [pos_x;
          pos_y;
          pos_z];
          % roll;
          % 0;
          % yaw];

pos_z_dot = 1 / 12;

% hover for 5 s
if (time < 5)
    pos_x_dot = 0;
    pos_y_dot = 0;
else
    pos_x_dot = - f * r * sin(arg);
    pos_y_dot = f * r * cos(arg);
end

% yaw_dot = 0;

pose_d_dot = [pos_x_dot;
              pos_y_dot;
              pos_z_dot];
              % 0;
              % 0;
              % yaw_dot];

pos_z_ddot = 0;
% hover for 5 s
if (time < 5)
    pos_x_ddot = 0;
    pos_y_ddot = 0;
else
    pos_x_ddot = - f * f * r * cos(arg);
    pos_y_ddot = - f * f * r * sin(arg);
end

% yaw_ddot = 0;

pose_d_ddot = [pos_x_ddot;
               pos_y_ddot;
               pos_z_ddot];
               % 0;
               % 0;
               % yaw_ddot];

== matlab function quad_6DOF_quaternion_ANSFT/Lemniscate Trajectory ==
  data: time input; pose_d output; pose_d_dot output; pose_d_ddot output
function [pose_d, pose_d_dot, pose_d_ddot]= fcn(time)

%% Positions

arg = time / 4;

pos_x = cos(arg) ./ (1 + sin(arg) .* sin(arg));
pos_y = cos(arg) .* sin(arg) ./ (1 + sin(arg) .* sin(arg));
pos_z = sin(arg);

% yaw = time * 0;

pose_d = [pos_x;
          pos_y;
          pos_z];
          % 0;
          % 0;
          % yaw];

%% Velocities

pos_z_dot = 0.25 * cos(arg);
pos_x_dot = - sin(arg)/(4*(sin(arg)^2 + 1)) - (cos(arg)^2*sin(arg))/(2*(sin(arg)^2 + 1)^2);
pos_y_dot = cos(arg)^2/(4*(sin(arg)^2 + 1)) - sin(arg)^2/(4*(sin(arg)^2 + 1)) - (cos(arg)^2*sin(arg)^2)/(2*(sin(arg)^2 + 1)^2);
% yaw_dot = 0;

pose_d_dot = [pos_x_dot;
              pos_y_dot;
              pos_z_dot];
              % 0;
              % 0;
              % yaw_dot];

%% Accelerations

pos_z_ddot = -0.25 * 0.25 * sin(arg);
pos_x_ddot = 0;
pos_y_ddot = 0;
% yaw_ddot = 0;

pose_d_ddot = [pos_x_ddot;
               pos_y_ddot;
               pos_z_ddot];
               % 0;
               % 0;
               % yaw_ddot];
